simulink model "wave_2"  (Simulink 7.4)
settings: Solver=ode23tb  StartTime=0.0  StopTime=.5  RelTol=1e-3
PreLoadFcn:
  | load gauss_fir;  % pulse shaping coefficients
InitFcn:
  | Ts=1e-4;    % set this to control simulation speed, mainly for wave visualization
  | Line_Length=.05; % in meters
libraries: powerlib x209, simulink x2, dspsrcs4 x1
(part 1 of 2)
settings Model: Creator=Dick  LastModifiedBy=Dick
settings SolverCC: SolverResetMethod=Robust
settings DebuggingCC: SolverPrmCheckMsg=none

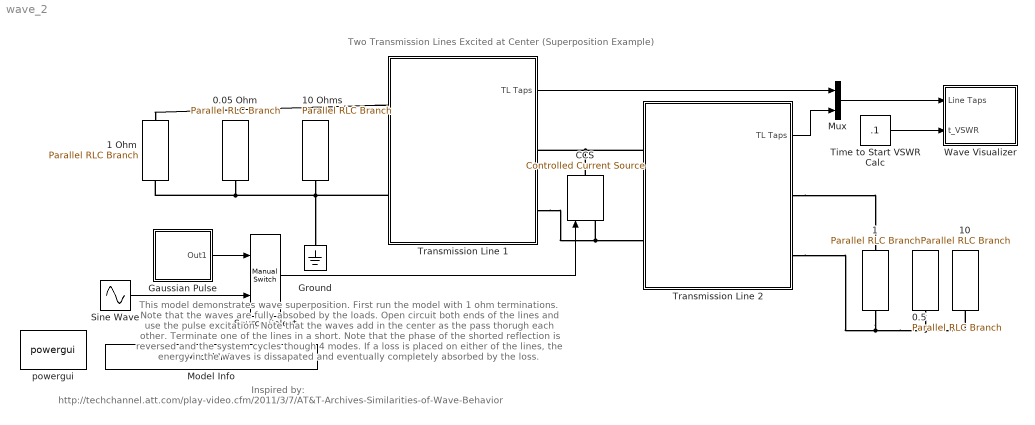
== system wave_2 ==
  note: Two Transmission Lines Excited at Center (Superposition Example)
  note: Inspired by: http://techchannel.att.com/play-video.cfm/2011/3/7/AT&T-Archives-Similarities-of-Wave-Behavior
  note: This model demonstrates wave superposition. First run the model with 1 ohm terminations. Note that the
      | waves are fully absobed by the loads. Open circuit both ends of the lines and use the pulse excitation.
      | Note that the waves add in the center as the pass thorugh each other.
      | Terminate one of the lines in a short. Note that the phase of the shorted reflection
      | is reversed and the system cycles though 4 modes. If a loss is placed on either of the lines,
      | the energy in the waves is dissapated and eventually completely absorbed by the loss.
  0.05 Ohm : powerlib/Elements/Parallel RLC Branch  DialogController=POWERSYS.PowerSysDialog  PhysicalDomain=powersysdomain  SubClassName=unknown  LeftPortType=p1  RightPortType=p1  LConnTagsString=a  RConnTagsString=__new0  BranchType=R  Resistance=.05  Inductance=1e-3  SetiL0=off  InitialCurrent=0  Capacitance=1  Setx0=off  InitialVoltage=0  Measurements=None
  0.5 : powerlib/Elements/Parallel RLC Branch  DialogController=POWERSYS.PowerSysDialog  PhysicalDomain=powersysdomain  SubClassName=unknown  LeftPortType=p1  RightPortType=p1  LConnTagsString=a  RConnTagsString=__new0  BranchType=R  Resistance=.05  Inductance=1e-3  SetiL0=off  InitialCurrent=0  Capacitance=1  Setx0=off  InitialVoltage=0  Measurements=None
  1 : powerlib/Elements/Parallel RLC Branch  DialogController=POWERSYS.PowerSysDialog  PhysicalDomain=powersysdomain  SubClassName=unknown  LeftPortType=p1  RightPortType=p1  LConnTagsString=a  RConnTagsString=__new0  BranchType=R  Resistance=1  Inductance=1e-3  SetiL0=off  InitialCurrent=0  Capacitance=1  Setx0=off  InitialVoltage=0  Measurements=None
  1 Ohm : powerlib/Elements/Parallel RLC Branch  DialogController=POWERSYS.PowerSysDialog  PhysicalDomain=powersysdomain  SubClassName=unknown  LeftPortType=p1  RightPortType=p1  LConnTagsString=a  RConnTagsString=__new0  BranchType=R  Resistance=1  Inductance=1e-3  SetiL0=off  InitialCurrent=0  Capacitance=1  Setx0=off  InitialVoltage=0  Measurements=None
  10 : powerlib/Elements/Parallel RLC Branch  DialogController=POWERSYS.PowerSysDialog  PhysicalDomain=powersysdomain  SubClassName=unknown  LeftPortType=p1  RightPortType=p1  LConnTagsString=a  RConnTagsString=__new0  BranchType=R  Resistance=10  Inductance=1e-3  SetiL0=off  InitialCurrent=0  Capacitance=1  Setx0=off  InitialVoltage=0  Measurements=None
  10 Ohms : powerlib/Elements/Parallel RLC Branch  DialogController=POWERSYS.PowerSysDialog  PhysicalDomain=powersysdomain  SubClassName=unknown  LeftPortType=p1  RightPortType=p1  LConnTagsString=a  RConnTagsString=__new0  BranchType=R  Resistance=10  Inductance=1e-3  SetiL0=off  InitialCurrent=0  Capacitance=1  Setx0=off  InitialVoltage=0  Measurements=None
  CCS : powerlib/Electrical Sources/Controlled Current Source  DialogController=POWERSYS.PowerSysDialog  SystemSampleTime=-1  Initialize=off  Source_Type=DC  Amplitude=0  Phase=0  Frequency=0  Measurements=None
  Gaussian Pulse : Subsystem
  Ground : powerlib/Elements/Ground  DialogController=POWERSYS.PowerSysDialog  PhysicalDomain=powersysdomain  SubClassName=unknown  LeftPortType=p1  RightPortType=p1  LConnTagsString=a
  Model Info : simulink/Model-Wide Utilities/Model Info  SystemSampleTime=-1  InitialBlockCM=None  BlockCM=None  Frame=on  DisplayStringWithTags=Copyright 2012 The MathWorks, Inc.  HorizontalTextAlignment=Center  LeftAlignmentValue=0.5  SourceBlockDiagram=wave_2  TagMaxNumber=20
  Mux : Mux  Inputs=2
  Sine Wave : Sin  Amplitude=1  Bias=0  Frequency=40*2*pi  Phase=0  Samples=10  SampleTime=Ts  Offset=0
  Source Select : simulink/Signal Routing/Manual Switch  SystemSampleTime=-1  sw=0  action=0  varsize=off
  Time to Start VSWR Calc : Constant  Value=.1  OutDataType=fixdt(1, 16)  OutScaling=2^0
  Transmission Line 1 : Subsystem  mask{Zo=1, Vp=1, Len=Line_Length}
      mask prompts: Zo "Zo in ohms"; Vp "Vp in meters/sec"; Len "Line Length in meters"
      mask init:
      | C_1 = ones(1,10)/(Vp*Zo);  % farads/meter
      | L_1 = ones(1,10)*Zo/Vp;    % henrys/meter
      mask CallbackString:
      | % C_1 = ones(1,10)/(Vp*Zo);  % farads/meter
      | % L_1 = ones(1,10)*Zo/Vp;    % henrys/meter
      | |%C_1 = ones(1,10)/(Vp*Zo);  % farads/meter
      | % L_1 = ones(1,10)*Zo/Vp;    % henrys/meter
      | |
      mask Display:
      | disp(['50 Tap Uniform\n Transmission Line \n\n',...
      |        'Zo=',num2str(Zo),' Ohms, \nVp=',num2str(Vp),'m/sec \n',...
      |        'Length=',num2str(Len),' meters'])
  Transmission Line 2 : Subsystem  mask{Zo=1, Vp=1, Len=Line_Length}
      mask prompts: Zo "Zo in ohms"; Vp "Vp in meters/sec"; Len "Line Length in meters"
      mask init:
      | C_1 = ones(1,10)/(Vp*Zo);  % farads/meter
      | L_1 = ones(1,10)*Zo/Vp;    % henrys/meter
      mask CallbackString:
      | % C_1 = ones(1,10)/(Vp*Zo);  % farads/meter
      | % L_1 = ones(1,10)*Zo/Vp;    % henrys/meter
      | |%C_1 = ones(1,10)/(Vp*Zo);  % farads/meter
      | % L_1 = ones(1,10)*Zo/Vp;    % henrys/meter
      | |
      mask Display:
      | disp(['50 Tap Uniform\n Transmission Line \n\n',...
      |        'Zo=',num2str(Zo),' Ohms, \nVp=',num2str(Vp),'m/sec \n',...
      |        'Length=',num2str(Len),' meters'])
  "Wave Visualizer " : Subsystem
  powergui : powerlib/powergui  Priority=1  SystemSampleTime=-1  SimulationMode=Continuous  SampleTime=50e-6  frequency=60  SPID=off  DisableSnubberDevices=off  DisableRonSwitches=off  DisableVfSwitches=off  SwTol=0  Interpol=off  frequencyindice=0  echomessages=off  HookPort=off  DisplayEquations=off  FunctionMessages=off  EnableUseOfTLC=off  x0status=blocks  RestoreLinks=warning  Frange=[0:2:500]  Ylog=off  Xlog=on  ShowGrid=off  save=off  variable=ZData  ZoomFFT=on  StartTime=0.0  cycles=1  DisplayStyle=1  fundamental=60  FreqAxis=off  MaxFrequency=1000  frequencyindicesteady=1  RmsSteady=1  display=off  Ts=0  methode=off
  wires:
  Sine Wave/1 -> Source Select/2
  Gaussian Pulse/1(Out1) -> Source Select/1
  Mux/1 -> "Wave Visualizer "/1(Line Taps)
  Transmission Line 1/1(TL Taps) -> Mux/1
  Transmission Line 2/1(TL Taps) -> Mux/2
  Time to Start VSWR Calc/1 -> "Wave Visualizer "/2(t_VSWR)
  Source Select/1 -> CCS/1
  connections:
  Transmission Line 1/LConn2 -- 0.05 Ohm/RConn1 -- 1 Ohm/RConn1 -- 10 Ohms/RConn1 -- Ground/LConn1
  Transmission Line 2/RConn2 -- 10/RConn1 -- 0.5/RConn1 -- 1/RConn1
  Transmission Line 2/LConn1 -- Transmission Line 1/RConn1 -- CCS/RConn1
  Transmission Line 1/RConn2 -- Transmission Line 2/LConn2 -- CCS/LConn1
  Transmission Line 1/LConn1 -- 1 Ohm/LConn1
  Transmission Line 2/RConn1 -- 1/LConn1

== system wave_2/Gaussian Pulse ==
  Discrete  Impulse : dspsrcs4/Discrete  Impulse  Delay=0  SampleTime=Ts  FrameSample=1  dataType=double  isSigned=on  wordLen=16  udDataType=sfix(16)  fracBitsMode=Best precision  numFracBits=15
  Discrete FIR Filter : DiscreteFir  NumCoeffs=h_gauss
  Out1 : Outport
  wires:
  Discrete  Impulse/1 -> Discrete FIR Filter/1
  Discrete FIR Filter/1 -> Out1/1

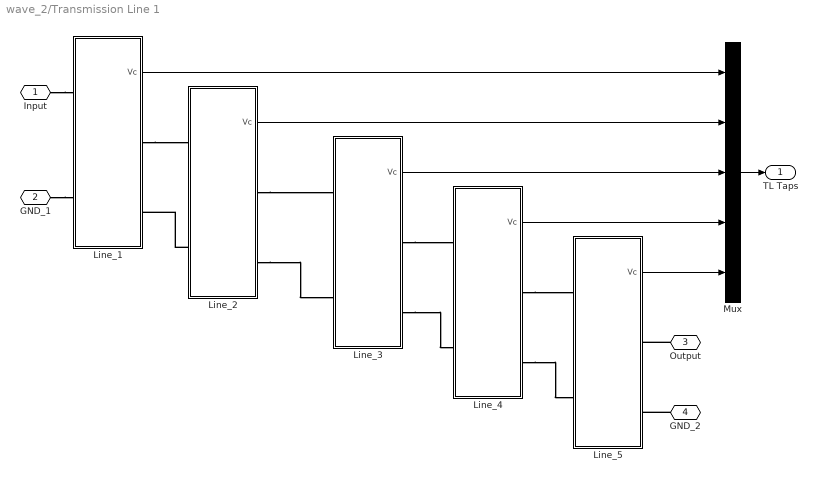
== system wave_2/Transmission Line 1 ==
  Line_1 : Subsystem  mask{R=zeros(1,10), L=L_1, C=C_1, Len=Len/5}
      mask prompts: R "Rvector(1:10) ohms/meter"; L "Lvector(1:10) henrys/meter"; C "Cvector(1:10) farards/meter"; Len "Length in m"
      mask Display: disp('TRL Section')
  Line_2 : Subsystem  mask{R=zeros(1,10), L=L_1, C=C_1, Len=Len/5}
      mask prompts: R "Rvector(1:10) ohms/meter"; L "Lvector(1:10) henrys/meter"; C "Cvector(1:10) farards/meter"; Len "Length in m"
      mask Display: disp('TRL Section')
  Line_3 : Subsystem  mask{R=zeros(1,10), L=L_1, C=C_1, Len=Len/5}
      mask prompts: R "Rvector(1:10) ohms/meter"; L "Lvector(1:10) henrys/meter"; C "Cvector(1:10) farards/meter"; Len "Length in m"
      mask Display: disp('TRL Section')
  Line_4 : Subsystem  mask{R=zeros(1,10), L=L_1, C=C_1, Len=Len/5}
      mask prompts: R "Rvector(1:10) ohms/meter"; L "Lvector(1:10) henrys/meter"; C "Cvector(1:10) farards/meter"; Len "Length in m"
      mask Display: disp('TRL Section')
  Line_5 : Subsystem  mask{R=zeros(1,10), L=L_1, C=C_1, Len=Len/5}
      mask prompts: R "Rvector(1:10) ohms/meter"; L "Lvector(1:10) henrys/meter"; C "Cvector(1:10) farards/meter"; Len "Length in m"
      mask Display: disp('TRL Section')
  Mux : Mux  Inputs=5
  Input : PMIOPort  Port=1  Side=Left
  GND_1 : PMIOPort  Port=2  Side=Left
  Output : PMIOPort  Port=3  Side=Right
  GND_2 : PMIOPort  Port=4  Side=Right
  TL Taps : Outport
  wires:
  Line_1/1(Vc) -> Mux/1
  Line_2/1(Vc) -> Mux/2
  Line_5/1(Vc) -> Mux/5
  Line_3/1(Vc) -> Mux/3
  Line_4/1(Vc) -> Mux/4
  Mux/1 -> TL Taps/1
  connections:
  Line_1/RConn1 -- Line_2/LConn1
  Line_2/LConn2 -- Line_1/RConn2
  Line_2/RConn1 -- Line_3/LConn1
  Line_2/RConn2 -- Line_3/LConn2
  Line_3/RConn1 -- Line_4/LConn1
  Line_3/RConn2 -- Line_4/LConn2
  Line_4/RConn1 -- Line_5/LConn1
  Line_4/RConn2 -- Line_5/LConn2
  Input/RConn1 -- Line_1/LConn1
  GND_1/RConn1 -- Line_1/LConn2
  Output/RConn1 -- Line_5/RConn1
  GND_2/RConn1 -- Line_5/RConn2

== system wave_2/Transmission Line 2 ==
  Line_1 : Subsystem  mask{R=zeros(1,10), L=L_1, C=C_1, Len=Len/5}
      mask prompts: R "Rvector(1:10) ohms/meter"; L "Lvector(1:10) henrys/meter"; C "Cvector(1:10) farards/meter"; Len "Length in m"
      mask Display: disp('TRL Section')
  Line_2 : Subsystem  mask{R=zeros(1,10), L=L_1, C=C_1, Len=Len/5}
      mask prompts: R "Rvector(1:10) ohms/meter"; L "Lvector(1:10) henrys/meter"; C "Cvector(1:10) farards/meter"; Len "Length in m"
      mask Display: disp('TRL Section')
  Line_3 : Subsystem  mask{R=zeros(1,10), L=L_1, C=C_1, Len=Len/5}
      mask prompts: R "Rvector(1:10) ohms/meter"; L "Lvector(1:10) henrys/meter"; C "Cvector(1:10) farards/meter"; Len "Length in m"
      mask Display: disp('TRL Section')
  Line_4 : Subsystem  mask{R=zeros(1,10), L=L_1, C=C_1, Len=Len/5}
      mask prompts: R "Rvector(1:10) ohms/meter"; L "Lvector(1:10) henrys/meter"; C "Cvector(1:10) farards/meter"; Len "Length in m"
      mask Display: disp('TRL Section')
  Line_5 : Subsystem  mask{R=zeros(1,10), L=L_1, C=C_1, Len=Len/5}
      mask prompts: R "Rvector(1:10) ohms/meter"; L "Lvector(1:10) henrys/meter"; C "Cvector(1:10) farards/meter"; Len "Length in m"
      mask Display: disp('TRL Section')
  Mux : Mux  Inputs=5
  Input : PMIOPort  Port=1  Side=Left
  GND_1 : PMIOPort  Port=2  Side=Left
  Output : PMIOPort  Port=3  Side=Right
  GND_2 : PMIOPort  Port=4  Side=Right
  TL Taps : Outport
  wires:
  Mux/1 -> TL Taps/1
  Line_4/1(Vc) -> Mux/4
  Line_3/1(Vc) -> Mux/3
  Line_5/1(Vc) -> Mux/5
  Line_2/1(Vc) -> Mux/2
  Line_1/1(Vc) -> Mux/1
  connections:
  GND_2/RConn1 -- Line_5/RConn2
  Output/RConn1 -- Line_5/RConn1
  GND_1/RConn1 -- Line_1/LConn2
  Input/RConn1 -- Line_1/LConn1
  Line_4/RConn2 -- Line_5/LConn2
  Line_4/RConn1 -- Line_5/LConn1
  Line_3/RConn2 -- Line_4/LConn2
  Line_3/RConn1 -- Line_4/LConn1
  Line_2/RConn2 -- Line_3/LConn2
  Line_2/RConn1 -- Line_3/LConn1
  Line_2/LConn2 -- Line_1/RConn2
  Line_1/RConn1 -- Line_2/LConn1

== system wave_2/Wave Visualizer  ==
  note: The VSWR calculaltion uses the maximum and minimum values of the PEAK of the wave over the simulation run.
      | Therefore, the transmision line system needs to have achieved steady state conditions before the calculation is started.
      | This time will vary with line configurations as well as source and load terminations. Ther VSWR is measured on Line 1.
      | Obviously the sine source must be used.
  Line Taps : Inport
  t_VSWR : Inport  Port=2
  Clock : Clock
  Constant3 : Constant  Value=Line_Length  OutDataType=fixdt(1, 16)  OutScaling=2^0  SampleTime=Ts
  Line  Section Tap  Voltage : Stateflow chart
  Zero-Order Hold : ZeroOrderHold  SampleTime=Ts
  Zero-Order Hold1 : ZeroOrderHold  SampleTime=Ts
  wires:
  Zero-Order Hold/1 -> Line  Section Tap  Voltage/1(y)
  Constant3/1 -> Line  Section Tap  Voltage/3(Line_Length)
  Clock/1 -> Zero-Order Hold1/1
  Zero-Order Hold1/1 -> Line  Section Tap  Voltage/2(t)
  Line Taps/1 -> Zero-Order Hold/1
  t_VSWR/1 -> Line  Section Tap  Voltage/4(t_VSWR)

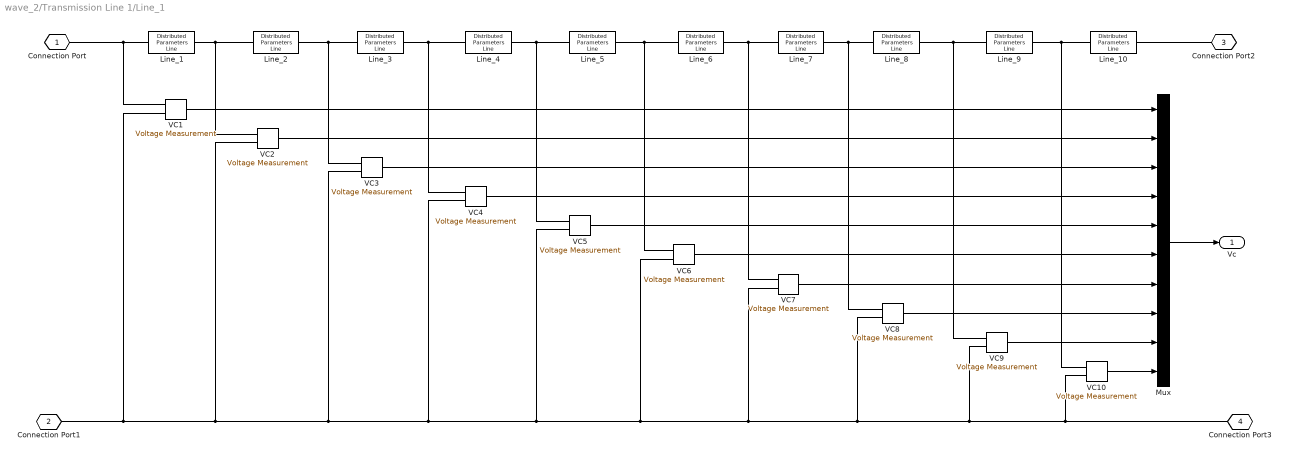
== system wave_2/Transmission Line 1/Line_1 ==
  Line_1 : powerlib/Elements/Distributed Parameters Line  DialogController=POWERSYS.PowerSysDialog  SystemSampleTime=-1  Phases=1  Frequency=60  Resistance=R(1)*1000  Inductance=L(1)*1000  Capacitance=C(1)*1000  Length=Len/(10*1000); % 10 sections in this subsystem  x1=[0 0;0.0002 0;0.0004 0;0.0006 0;0.0008 0;0.001 0]  x2=[0 0;0.0002 0;0.0004 0;0.0006 0;0.0008 0;0.001 0]  x3=[0 0;0.0002 0;0.0004 0;0.0006 0;0.0008 0;0.001 0]  x4=[0 0;0.0002 0;0.0004 0;0.0006 0;0.0008 0;0.001 0]  x5=0.001  Measurements=None
  Line_10 : powerlib/Elements/Distributed Parameters Line  DialogController=POWERSYS.PowerSysDialog  SystemSampleTime=-1  Phases=1  Frequency=60  Resistance=R(10)*1000  Inductance=L(10)*1000  Capacitance=C(10)*1000  Length=Len/(10*1000); % 10 sections in this subsystem  x1=[0 0;0.0002 0;0.0004 0;0.0006 0;0.0008 0;0.001 0]  x2=[0 0;0.0002 0;0.0004 0;0.0006 0;0.0008 0;0.001 0]  x3=[0 0;0.0002 0;0.0004 0;0.0006 0;0.0008 0;0.001 0]  x4=[0 0;0.0002 0;0.0004 0;0.0006 0;0.0008 0;0.001 0]  x5=0.001  Measurements=None
  Line_2 : powerlib/Elements/Distributed Parameters Line  DialogController=POWERSYS.PowerSysDialog  SystemSampleTime=-1  Phases=1  Frequency=60  Resistance=R(2)*1000  Inductance=L(2)*1000  Capacitance=C(2)*1000  Length=Len/(10*1000); % 10 sections in this subsystem  x1=[0 0;0.0002 0;0.0004 0;0.0006 0;0.0008 0;0.001 0]  x2=[0 0;0.0002 0;0.0004 0;0.0006 0;0.0008 0;0.001 0]  x3=[0 0;0.0002 0;0.0004 0;0.0006 0;0.0008 0;0.001 0]  x4=[0 0;0.0002 0;0.0004 0;0.0006 0;0.0008 0;0.001 0]  x5=0.001  Measurements=None
  Line_3 : powerlib/Elements/Distributed Parameters Line  DialogController=POWERSYS.PowerSysDialog  SystemSampleTime=-1  Phases=1  Frequency=60  Resistance=R(3)*1000  Inductance=L(3)*1000  Capacitance=C(3)*1000  Length=Len/(10*1000); % 10 sections in this subsystem  x1=[0 0;0.0002 0;0.0004 0;0.0006 0;0.0008 0;0.001 0]  x2=[0 0;0.0002 0;0.0004 0;0.0006 0;0.0008 0;0.001 0]  x3=[0 0;0.0002 0;0.0004 0;0.0006 0;0.0008 0;0.001 0]  x4=[0 0;0.0002 0;0.0004 0;0.0006 0;0.0008 0;0.001 0]  x5=0.001  Measurements=None
  Line_4 : powerlib/Elements/Distributed Parameters Line  DialogController=POWERSYS.PowerSysDialog  SystemSampleTime=-1  Phases=1  Frequency=60  Resistance=R(4)*1000  Inductance=L(4)*1000  Capacitance=C(4)*1000  Length=Len/(10*1000); % 10 sections in this subsystem  x1=[0 0;0.0002 0;0.0004 0;0.0006 0;0.0008 0;0.001 0]  x2=[0 0;0.0002 0;0.0004 0;0.0006 0;0.0008 0;0.001 0]  x3=[0 0;0.0002 0;0.0004 0;0.0006 0;0.0008 0;0.001 0]  x4=[0 0;0.0002 0;0.0004 0;0.0006 0;0.0008 0;0.001 0]  x5=0.001  Measurements=None
  Line_5 : powerlib/Elements/Distributed Parameters Line  DialogController=POWERSYS.PowerSysDialog  SystemSampleTime=-1  Phases=1  Frequency=60  Resistance=R(5)*1000  Inductance=L(5)*1000  Capacitance=C(5)*1000  Length=Len/(10*1000); % 10 sections in this subsystem  x1=[0 0;0.0002 0;0.0004 0;0.0006 0;0.0008 0;0.001 0]  x2=[0 0;0.0002 0;0.0004 0;0.0006 0;0.0008 0;0.001 0]  x3=[0 0;0.0002 0;0.0004 0;0.0006 0;0.0008 0;0.001 0]  x4=[0 0;0.0002 0;0.0004 0;0.0006 0;0.0008 0;0.001 0]  x5=0.001  Measurements=None
  Line_6 : powerlib/Elements/Distributed Parameters Line  DialogController=POWERSYS.PowerSysDialog  SystemSampleTime=-1  Phases=1  Frequency=60  Resistance=R(6)*1000  Inductance=L(6)*1000  Capacitance=C(6)*1000  Length=Len/(10*1000); % 10 sections in this subsystem  x1=[0 0;0.0002 0;0.0004 0;0.0006 0;0.0008 0;0.001 0]  x2=[0 0;0.0002 0;0.0004 0;0.0006 0;0.0008 0;0.001 0]  x3=[0 0;0.0002 0;0.0004 0;0.0006 0;0.0008 0;0.001 0]  x4=[0 0;0.0002 0;0.0004 0;0.0006 0;0.0008 0;0.001 0]  x5=0.001  Measurements=None
  Line_7 : powerlib/Elements/Distributed Parameters Line  DialogController=POWERSYS.PowerSysDialog  SystemSampleTime=-1  Phases=1  Frequency=60  Resistance=R(7)*1000  Inductance=L(7)*1000  Capacitance=C(7)*1000  Length=Len/(10*1000); % 10 sections in this subsystem  x1=[0 0;0.0002 0;0.0004 0;0.0006 0;0.0008 0;0.001 0]  x2=[0 0;0.0002 0;0.0004 0;0.0006 0;0.0008 0;0.001 0]  x3=[0 0;0.0002 0;0.0004 0;0.0006 0;0.0008 0;0.001 0]  x4=[0 0;0.0002 0;0.0004 0;0.0006 0;0.0008 0;0.001 0]  x5=0.001  Measurements=None
  Line_8 : powerlib/Elements/Distributed Parameters Line  DialogController=POWERSYS.PowerSysDialog  SystemSampleTime=-1  Phases=1  Frequency=60  Resistance=R(8)*1000  Inductance=L(8)*1000  Capacitance=C(8)*1000  Length=Len/(10*1000); % 10 sections in this subsystem  x1=[0 0;0.0002 0;0.0004 0;0.0006 0;0.0008 0;0.001 0]  x2=[0 0;0.0002 0;0.0004 0;0.0006 0;0.0008 0;0.001 0]  x3=[0 0;0.0002 0;0.0004 0;0.0006 0;0.0008 0;0.001 0]  x4=[0 0;0.0002 0;0.0004 0;0.0006 0;0.0008 0;0.001 0]  x5=0.001  Measurements=None
  Line_9 : powerlib/Elements/Distributed Parameters Line  DialogController=POWERSYS.PowerSysDialog  SystemSampleTime=-1  Phases=1  Frequency=60  Resistance=R(9)*1000  Inductance=L(9)*1000  Capacitance=C(9)*1000  Length=Len/(10*1000); % 10 sections in this subsystem  x1=[0 0;0.0002 0;0.0004 0;0.0006 0;0.0008 0;0.001 0]  x2=[0 0;0.0002 0;0.0004 0;0.0006 0;0.0008 0;0.001 0]  x3=[0 0;0.0002 0;0.0004 0;0.0006 0;0.0008 0;0.001 0]  x4=[0 0;0.0002 0;0.0004 0;0.0006 0;0.0008 0;0.001 0]  x5=0.001  Measurements=None
  Mux : Mux  Inputs=10
  VC{1..10} (10 alike) : powerlib/Measurements/Voltage Measurement  DialogController=POWERSYS.PowerSysDialog  SystemSampleTime=-1  PhasorSimulation=off  OutputType=Complex  PSBequivalent=0
  Connection Port : PMIOPort  Tag=PMCPort  Port=1  Side=Left
  Connection Port1 : PMIOPort  Tag=PMCPort  Port=2  Side=Left
  Connection Port2 : PMIOPort  Tag=PMCPort  Port=3  Side=Right
  Connection Port3 : PMIOPort  Tag=PMCPort  Port=4  Side=Right
  Vc : Outport  OutDataType=fixdt(1, 16)  OutScaling=2^0
  wires:
  VC1/1 -> Mux/1
  VC10/1 -> Mux/10
  VC9/1 -> Mux/9
  VC8/1 -> Mux/8
  VC7/1 -> Mux/7
  VC6/1 -> Mux/6
  VC5/1 -> Mux/5
  VC4/1 -> Mux/4
  VC3/1 -> Mux/3
  VC2/1 -> Mux/2
  Mux/1 -> Vc/1
  connections:
  Connection Port1/RConn1 -- Connection Port3/RConn1 -- VC10/LConn2 -- VC9/LConn2 -- VC8/LConn2 -- VC7/LConn2 -- VC6/LConn2 -- VC5/LConn2 -- VC4/LConn2 -- VC3/LConn2 -- VC2/LConn2 -- VC1/LConn2
  Line_10/RConn1 -- Connection Port2/RConn1
  Connection Port/RConn1 -- Line_1/LConn1 -- VC1/LConn1
  Line_1/RConn1 -- Line_2/LConn1 -- VC2/LConn1
  Line_2/RConn1 -- Line_3/LConn1 -- VC3/LConn1
  Line_3/RConn1 -- Line_4/LConn1 -- VC4/LConn1
  Line_4/RConn1 -- Line_5/LConn1 -- VC5/LConn1
  Line_5/RConn1 -- Line_6/LConn1 -- VC6/LConn1
  Line_6/RConn1 -- Line_7/LConn1 -- VC7/LConn1
  Line_7/RConn1 -- Line_8/LConn1 -- VC8/LConn1
  Line_8/RConn1 -- Line_9/LConn1 -- VC9/LConn1
  Line_9/RConn1 -- Line_10/LConn1 -- VC10/LConn1

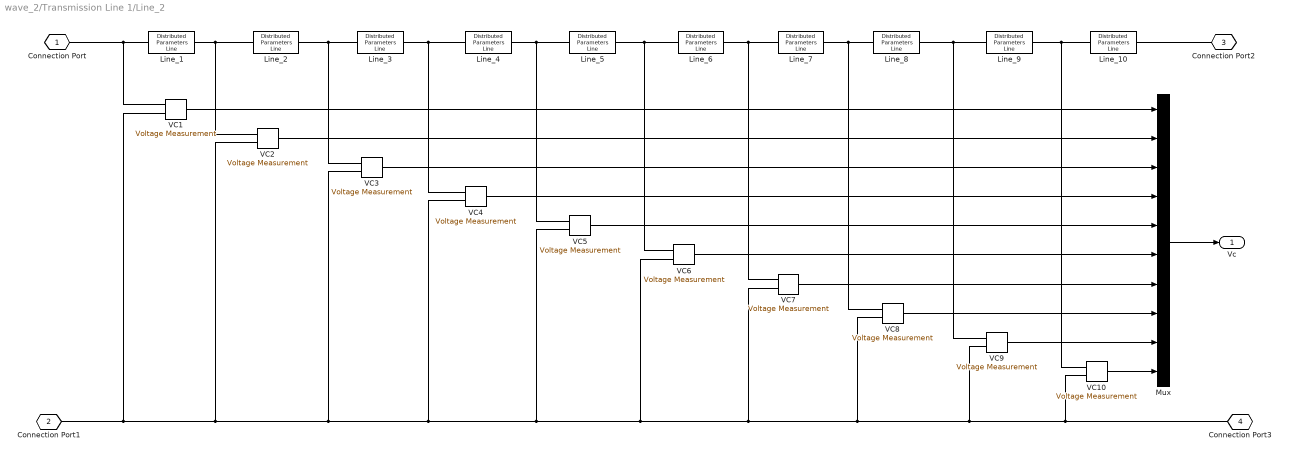
== system wave_2/Transmission Line 1/Line_2 ==
  Line_1 : powerlib/Elements/Distributed Parameters Line  DialogController=POWERSYS.PowerSysDialog  SystemSampleTime=-1  Phases=1  Frequency=60  Resistance=R(1)*1000  Inductance=L(1)*1000  Capacitance=C(1)*1000  Length=Len/(10*1000); % 10 sections in this subsystem  x1=[0 0;0.0002 0;0.0004 0;0.0006 0;0.0008 0;0.001 0]  x2=[0 0;0.0002 0;0.0004 0;0.0006 0;0.0008 0;0.001 0]  x3=[0 0;0.0002 0;0.0004 0;0.0006 0;0.0008 0;0.001 0]  x4=[0 0;0.0002 0;0.0004 0;0.0006 0;0.0008 0;0.001 0]  x5=0.001  Measurements=None
  Line_10 : powerlib/Elements/Distributed Parameters Line  DialogController=POWERSYS.PowerSysDialog  SystemSampleTime=-1  Phases=1  Frequency=60  Resistance=R(10)*1000  Inductance=L(10)*1000  Capacitance=C(10)*1000  Length=Len/(10*1000); % 10 sections in this subsystem  x1=[0 0;0.0002 0;0.0004 0;0.0006 0;0.0008 0;0.001 0]  x2=[0 0;0.0002 0;0.0004 0;0.0006 0;0.0008 0;0.001 0]  x3=[0 0;0.0002 0;0.0004 0;0.0006 0;0.0008 0;0.001 0]  x4=[0 0;0.0002 0;0.0004 0;0.0006 0;0.0008 0;0.001 0]  x5=0.001  Measurements=None
  Line_2 : powerlib/Elements/Distributed Parameters Line  DialogController=POWERSYS.PowerSysDialog  SystemSampleTime=-1  Phases=1  Frequency=60  Resistance=R(2)*1000  Inductance=L(2)*1000  Capacitance=C(2)*1000  Length=Len/(10*1000); % 10 sections in this subsystem  x1=[0 0;0.0002 0;0.0004 0;0.0006 0;0.0008 0;0.001 0]  x2=[0 0;0.0002 0;0.0004 0;0.0006 0;0.0008 0;0.001 0]  x3=[0 0;0.0002 0;0.0004 0;0.0006 0;0.0008 0;0.001 0]  x4=[0 0;0.0002 0;0.0004 0;0.0006 0;0.0008 0;0.001 0]  x5=0.001  Measurements=None
  Line_3 : powerlib/Elements/Distributed Parameters Line  DialogController=POWERSYS.PowerSysDialog  SystemSampleTime=-1  Phases=1  Frequency=60  Resistance=R(3)*1000  Inductance=L(3)*1000  Capacitance=C(3)*1000  Length=Len/(10*1000); % 10 sections in this subsystem  x1=[0 0;0.0002 0;0.0004 0;0.0006 0;0.0008 0;0.001 0]  x2=[0 0;0.0002 0;0.0004 0;0.0006 0;0.0008 0;0.001 0]  x3=[0 0;0.0002 0;0.0004 0;0.0006 0;0.0008 0;0.001 0]  x4=[0 0;0.0002 0;0.0004 0;0.0006 0;0.0008 0;0.001 0]  x5=0.001  Measurements=None
  Line_4 : powerlib/Elements/Distributed Parameters Line  DialogController=POWERSYS.PowerSysDialog  SystemSampleTime=-1  Phases=1  Frequency=60  Resistance=R(4)*1000  Inductance=L(4)*1000  Capacitance=C(4)*1000  Length=Len/(10*1000); % 10 sections in this subsystem  x1=[0 0;0.0002 0;0.0004 0;0.0006 0;0.0008 0;0.001 0]  x2=[0 0;0.0002 0;0.0004 0;0.0006 0;0.0008 0;0.001 0]  x3=[0 0;0.0002 0;0.0004 0;0.0006 0;0.0008 0;0.001 0]  x4=[0 0;0.0002 0;0.0004 0;0.0006 0;0.0008 0;0.001 0]  x5=0.001  Measurements=None
  Line_5 : powerlib/Elements/Distributed Parameters Line  DialogController=POWERSYS.PowerSysDialog  SystemSampleTime=-1  Phases=1  Frequency=60  Resistance=R(5)*1000  Inductance=L(5)*1000  Capacitance=C(5)*1000  Length=Len/(10*1000); % 10 sections in this subsystem  x1=[0 0;0.0002 0;0.0004 0;0.0006 0;0.0008 0;0.001 0]  x2=[0 0;0.0002 0;0.0004 0;0.0006 0;0.0008 0;0.001 0]  x3=[0 0;0.0002 0;0.0004 0;0.0006 0;0.0008 0;0.001 0]  x4=[0 0;0.0002 0;0.0004 0;0.0006 0;0.0008 0;0.001 0]  x5=0.001  Measurements=None
  Line_6 : powerlib/Elements/Distributed Parameters Line  DialogController=POWERSYS.PowerSysDialog  SystemSampleTime=-1  Phases=1  Frequency=60  Resistance=R(6)*1000  Inductance=L(6)*1000  Capacitance=C(6)*1000  Length=Len/(10*1000); % 10 sections in this subsystem  x1=[0 0;0.0002 0;0.0004 0;0.0006 0;0.0008 0;0.001 0]  x2=[0 0;0.0002 0;0.0004 0;0.0006 0;0.0008 0;0.001 0]  x3=[0 0;0.0002 0;0.0004 0;0.0006 0;0.0008 0;0.001 0]  x4=[0 0;0.0002 0;0.0004 0;0.0006 0;0.0008 0;0.001 0]  x5=0.001  Measurements=None
  Line_7 : powerlib/Elements/Distributed Parameters Line  DialogController=POWERSYS.PowerSysDialog  SystemSampleTime=-1  Phases=1  Frequency=60  Resistance=R(7)*1000  Inductance=L(7)*1000  Capacitance=C(7)*1000  Length=Len/(10*1000); % 10 sections in this subsystem  x1=[0 0;0.0002 0;0.0004 0;0.0006 0;0.0008 0;0.001 0]  x2=[0 0;0.0002 0;0.0004 0;0.0006 0;0.0008 0;0.001 0]  x3=[0 0;0.0002 0;0.0004 0;0.0006 0;0.0008 0;0.001 0]  x4=[0 0;0.0002 0;0.0004 0;0.0006 0;0.0008 0;0.001 0]  x5=0.001  Measurements=None
  Line_8 : powerlib/Elements/Distributed Parameters Line  DialogController=POWERSYS.PowerSysDialog  SystemSampleTime=-1  Phases=1  Frequency=60  Resistance=R(8)*1000  Inductance=L(8)*1000  Capacitance=C(8)*1000  Length=Len/(10*1000); % 10 sections in this subsystem  x1=[0 0;0.0002 0;0.0004 0;0.0006 0;0.0008 0;0.001 0]  x2=[0 0;0.0002 0;0.0004 0;0.0006 0;0.0008 0;0.001 0]  x3=[0 0;0.0002 0;0.0004 0;0.0006 0;0.0008 0;0.001 0]  x4=[0 0;0.0002 0;0.0004 0;0.0006 0;0.0008 0;0.001 0]  x5=0.001  Measurements=None
  Line_9 : powerlib/Elements/Distributed Parameters Line  DialogController=POWERSYS.PowerSysDialog  SystemSampleTime=-1  Phases=1  Frequency=60  Resistance=R(9)*1000  Inductance=L(9)*1000  Capacitance=C(9)*1000  Length=Len/(10*1000); % 10 sections in this subsystem  x1=[0 0;0.0002 0;0.0004 0;0.0006 0;0.0008 0;0.001 0]  x2=[0 0;0.0002 0;0.0004 0;0.0006 0;0.0008 0;0.001 0]  x3=[0 0;0.0002 0;0.0004 0;0.0006 0;0.0008 0;0.001 0]  x4=[0 0;0.0002 0;0.0004 0;0.0006 0;0.0008 0;0.001 0]  x5=0.001  Measurements=None
  Mux : Mux  Inputs=10
  VC{1..10} (10 alike) : powerlib/Measurements/Voltage Measurement  DialogController=POWERSYS.PowerSysDialog  SystemSampleTime=-1  PhasorSimulation=off  OutputType=Complex  PSBequivalent=0
  Connection Port : PMIOPort  Tag=PMCPort  Port=1  Side=Left
  Connection Port1 : PMIOPort  Tag=PMCPort  Port=2  Side=Left
  Connection Port2 : PMIOPort  Tag=PMCPort  Port=3  Side=Right
  Connection Port3 : PMIOPort  Tag=PMCPort  Port=4  Side=Right
  Vc : Outport  OutDataType=fixdt(1, 16)  OutScaling=2^0
  wires:
  Mux/1 -> Vc/1
  VC2/1 -> Mux/2
  VC3/1 -> Mux/3
  VC4/1 -> Mux/4
  VC5/1 -> Mux/5
  VC6/1 -> Mux/6
  VC7/1 -> Mux/7
  VC8/1 -> Mux/8
  VC9/1 -> Mux/9
  VC10/1 -> Mux/10
  VC1/1 -> Mux/1
  connections:
  VC10/LConn1 -- Line_10/LConn1 -- Line_9/RConn1
  VC9/LConn1 -- Line_9/LConn1 -- Line_8/RConn1
  VC8/LConn1 -- Line_8/LConn1 -- Line_7/RConn1
  VC7/LConn1 -- Line_7/LConn1 -- Line_6/RConn1
  VC6/LConn1 -- Line_6/LConn1 -- Line_5/RConn1
  VC5/LConn1 -- Line_5/LConn1 -- Line_4/RConn1
  VC4/LConn1 -- Line_4/LConn1 -- Line_3/RConn1
  VC3/LConn1 -- Line_3/LConn1 -- Line_2/RConn1
  VC2/LConn1 -- Line_2/LConn1 -- Line_1/RConn1
  VC1/LConn1 -- Line_1/LConn1 -- Connection Port/RConn1
  Line_10/RConn1 -- Connection Port2/RConn1
  VC1/LConn2 -- VC2/LConn2 -- VC3/LConn2 -- VC4/LConn2 -- VC5/LConn2 -- VC6/LConn2 -- VC7/LConn2 -- VC8/LConn2 -- VC9/LConn2 -- VC10/LConn2 -- Connection Port3/RConn1 -- Connection Port1/RConn1

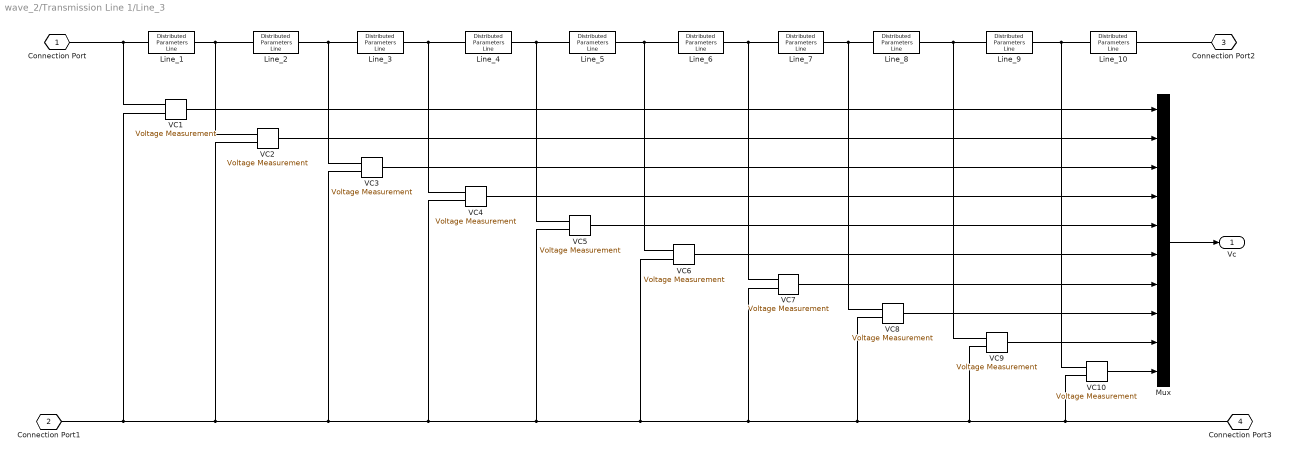
== system wave_2/Transmission Line 1/Line_3 ==
  Line_1 : powerlib/Elements/Distributed Parameters Line  DialogController=POWERSYS.PowerSysDialog  SystemSampleTime=-1  Phases=1  Frequency=60  Resistance=R(1)*1000  Inductance=L(1)*1000  Capacitance=C(1)*1000  Length=Len/(10*1000); % 10 sections in this subsystem  x1=[0 0;0.0002 0;0.0004 0;0.0006 0;0.0008 0;0.001 0]  x2=[0 0;0.0002 0;0.0004 0;0.0006 0;0.0008 0;0.001 0]  x3=[0 0;0.0002 0;0.0004 0;0.0006 0;0.0008 0;0.001 0]  x4=[0 0;0.0002 0;0.0004 0;0.0006 0;0.0008 0;0.001 0]  x5=0.001  Measurements=None
  Line_10 : powerlib/Elements/Distributed Parameters Line  DialogController=POWERSYS.PowerSysDialog  SystemSampleTime=-1  Phases=1  Frequency=60  Resistance=R(10)*1000  Inductance=L(10)*1000  Capacitance=C(10)*1000  Length=Len/(10*1000); % 10 sections in this subsystem  x1=[0 0;0.0002 0;0.0004 0;0.0006 0;0.0008 0;0.001 0]  x2=[0 0;0.0002 0;0.0004 0;0.0006 0;0.0008 0;0.001 0]  x3=[0 0;0.0002 0;0.0004 0;0.0006 0;0.0008 0;0.001 0]  x4=[0 0;0.0002 0;0.0004 0;0.0006 0;0.0008 0;0.001 0]  x5=0.001  Measurements=None
  Line_2 : powerlib/Elements/Distributed Parameters Line  DialogController=POWERSYS.PowerSysDialog  SystemSampleTime=-1  Phases=1  Frequency=60  Resistance=R(2)*1000  Inductance=L(2)*1000  Capacitance=C(2)*1000  Length=Len/(10*1000); % 10 sections in this subsystem  x1=[0 0;0.0002 0;0.0004 0;0.0006 0;0.0008 0;0.001 0]  x2=[0 0;0.0002 0;0.0004 0;0.0006 0;0.0008 0;0.001 0]  x3=[0 0;0.0002 0;0.0004 0;0.0006 0;0.0008 0;0.001 0]  x4=[0 0;0.0002 0;0.0004 0;0.0006 0;0.0008 0;0.001 0]  x5=0.001  Measurements=None
  Line_3 : powerlib/Elements/Distributed Parameters Line  DialogController=POWERSYS.PowerSysDialog  SystemSampleTime=-1  Phases=1  Frequency=60  Resistance=R(3)*1000  Inductance=L(3)*1000  Capacitance=C(3)*1000  Length=Len/(10*1000); % 10 sections in this subsystem  x1=[0 0;0.0002 0;0.0004 0;0.0006 0;0.0008 0;0.001 0]  x2=[0 0;0.0002 0;0.0004 0;0.0006 0;0.0008 0;0.001 0]  x3=[0 0;0.0002 0;0.0004 0;0.0006 0;0.0008 0;0.001 0]  x4=[0 0;0.0002 0;0.0004 0;0.0006 0;0.0008 0;0.001 0]  x5=0.001  Measurements=None
  Line_4 : powerlib/Elements/Distributed Parameters Line  DialogController=POWERSYS.PowerSysDialog  SystemSampleTime=-1  Phases=1  Frequency=60  Resistance=R(4)*1000  Inductance=L(4)*1000  Capacitance=C(4)*1000  Length=Len/(10*1000); % 10 sections in this subsystem  x1=[0 0;0.0002 0;0.0004 0;0.0006 0;0.0008 0;0.001 0]  x2=[0 0;0.0002 0;0.0004 0;0.0006 0;0.0008 0;0.001 0]  x3=[0 0;0.0002 0;0.0004 0;0.0006 0;0.0008 0;0.001 0]  x4=[0 0;0.0002 0;0.0004 0;0.0006 0;0.0008 0;0.001 0]  x5=0.001  Measurements=None
  Line_5 : powerlib/Elements/Distributed Parameters Line  DialogController=POWERSYS.PowerSysDialog  SystemSampleTime=-1  Phases=1  Frequency=60  Resistance=R(5)*1000  Inductance=L(5)*1000  Capacitance=C(5)*1000  Length=Len/(10*1000); % 10 sections in this subsystem  x1=[0 0;0.0002 0;0.0004 0;0.0006 0;0.0008 0;0.001 0]  x2=[0 0;0.0002 0;0.0004 0;0.0006 0;0.0008 0;0.001 0]  x3=[0 0;0.0002 0;0.0004 0;0.0006 0;0.0008 0;0.001 0]  x4=[0 0;0.0002 0;0.0004 0;0.0006 0;0.0008 0;0.001 0]  x5=0.001  Measurements=None
  Line_6 : powerlib/Elements/Distributed Parameters Line  DialogController=POWERSYS.PowerSysDialog  SystemSampleTime=-1  Phases=1  Frequency=60  Resistance=R(6)*1000  Inductance=L(6)*1000  Capacitance=C(6)*1000  Length=Len/(10*1000); % 10 sections in this subsystem  x1=[0 0;0.0002 0;0.0004 0;0.0006 0;0.0008 0;0.001 0]  x2=[0 0;0.0002 0;0.0004 0;0.0006 0;0.0008 0;0.001 0]  x3=[0 0;0.0002 0;0.0004 0;0.0006 0;0.0008 0;0.001 0]  x4=[0 0;0.0002 0;0.0004 0;0.0006 0;0.0008 0;0.001 0]  x5=0.001  Measurements=None
  Line_7 : powerlib/Elements/Distributed Parameters Line  DialogController=POWERSYS.PowerSysDialog  SystemSampleTime=-1  Phases=1  Frequency=60  Resistance=R(7)*1000  Inductance=L(7)*1000  Capacitance=C(7)*1000  Length=Len/(10*1000); % 10 sections in this subsystem  x1=[0 0;0.0002 0;0.0004 0;0.0006 0;0.0008 0;0.001 0]  x2=[0 0;0.0002 0;0.0004 0;0.0006 0;0.0008 0;0.001 0]  x3=[0 0;0.0002 0;0.0004 0;0.0006 0;0.0008 0;0.001 0]  x4=[0 0;0.0002 0;0.0004 0;0.0006 0;0.0008 0;0.001 0]  x5=0.001  Measurements=None
  Line_8 : powerlib/Elements/Distributed Parameters Line  DialogController=POWERSYS.PowerSysDialog  SystemSampleTime=-1  Phases=1  Frequency=60  Resistance=R(8)*1000  Inductance=L(8)*1000  Capacitance=C(8)*1000  Length=Len/(10*1000); % 10 sections in this subsystem  x1=[0 0;0.0002 0;0.0004 0;0.0006 0;0.0008 0;0.001 0]  x2=[0 0;0.0002 0;0.0004 0;0.0006 0;0.0008 0;0.001 0]  x3=[0 0;0.0002 0;0.0004 0;0.0006 0;0.0008 0;0.001 0]  x4=[0 0;0.0002 0;0.0004 0;0.0006 0;0.0008 0;0.001 0]  x5=0.001  Measurements=None
  Line_9 : powerlib/Elements/Distributed Parameters Line  DialogController=POWERSYS.PowerSysDialog  SystemSampleTime=-1  Phases=1  Frequency=60  Resistance=R(9)*1000  Inductance=L(9)*1000  Capacitance=C(9)*1000  Length=Len/(10*1000); % 10 sections in this subsystem  x1=[0 0;0.0002 0;0.0004 0;0.0006 0;0.0008 0;0.001 0]  x2=[0 0;0.0002 0;0.0004 0;0.0006 0;0.0008 0;0.001 0]  x3=[0 0;0.0002 0;0.0004 0;0.0006 0;0.0008 0;0.001 0]  x4=[0 0;0.0002 0;0.0004 0;0.0006 0;0.0008 0;0.001 0]  x5=0.001  Measurements=None
  Mux : Mux  Inputs=10
  VC{1..10} (10 alike) : powerlib/Measurements/Voltage Measurement  DialogController=POWERSYS.PowerSysDialog  SystemSampleTime=-1  PhasorSimulation=off  OutputType=Complex  PSBequivalent=0
  Connection Port : PMIOPort  Tag=PMCPort  Port=1  Side=Left
  Connection Port1 : PMIOPort  Tag=PMCPort  Port=2  Side=Left
  Connection Port2 : PMIOPort  Tag=PMCPort  Port=3  Side=Right
  Connection Port3 : PMIOPort  Tag=PMCPort  Port=4  Side=Right
  Vc : Outport  OutDataType=fixdt(1, 16)  OutScaling=2^0
  wires:
  VC1/1 -> Mux/1
  VC10/1 -> Mux/10
  VC9/1 -> Mux/9
  VC8/1 -> Mux/8
  VC7/1 -> Mux/7
  VC6/1 -> Mux/6
  VC5/1 -> Mux/5
  VC4/1 -> Mux/4
  VC3/1 -> Mux/3
  VC2/1 -> Mux/2
  Mux/1 -> Vc/1
  connections:
  Connection Port1/RConn1 -- Connection Port3/RConn1 -- VC10/LConn2 -- VC9/LConn2 -- VC8/LConn2 -- VC7/LConn2 -- VC6/LConn2 -- VC5/LConn2 -- VC4/LConn2 -- VC3/LConn2 -- VC2/LConn2 -- VC1/LConn2
  Line_10/RConn1 -- Connection Port2/RConn1
  Connection Port/RConn1 -- Line_1/LConn1 -- VC1/LConn1
  Line_1/RConn1 -- Line_2/LConn1 -- VC2/LConn1
  Line_2/RConn1 -- Line_3/LConn1 -- VC3/LConn1
  Line_3/RConn1 -- Line_4/LConn1 -- VC4/LConn1
  Line_4/RConn1 -- Line_5/LConn1 -- VC5/LConn1
  Line_5/RConn1 -- Line_6/LConn1 -- VC6/LConn1
  Line_6/RConn1 -- Line_7/LConn1 -- VC7/LConn1
  Line_7/RConn1 -- Line_8/LConn1 -- VC8/LConn1
  Line_8/RConn1 -- Line_9/LConn1 -- VC9/LConn1
  Line_9/RConn1 -- Line_10/LConn1 -- VC10/LConn1

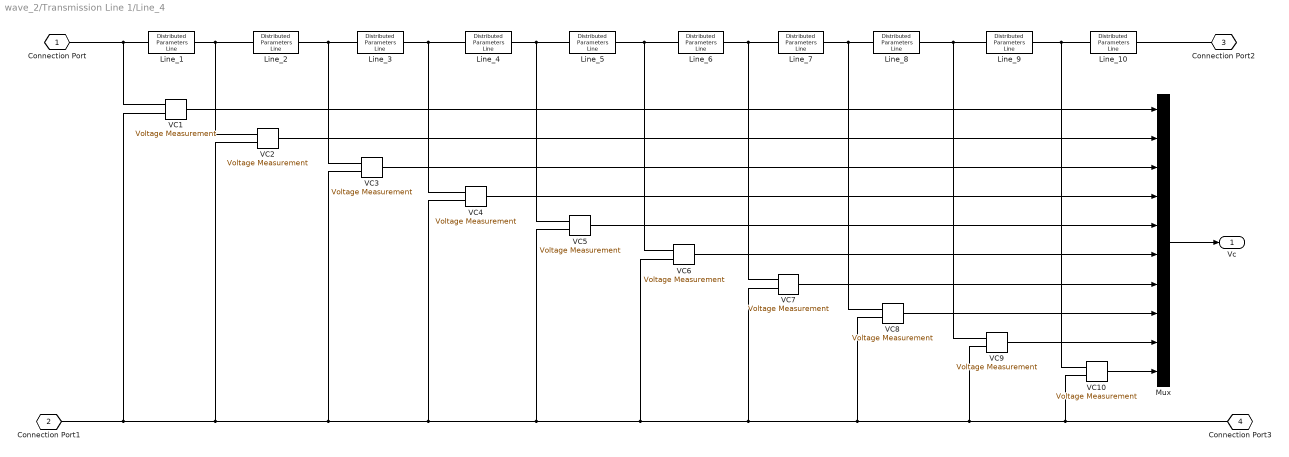
== system wave_2/Transmission Line 1/Line_4 ==
  Line_1 : powerlib/Elements/Distributed Parameters Line  DialogController=POWERSYS.PowerSysDialog  SystemSampleTime=-1  Phases=1  Frequency=60  Resistance=R(1)*1000  Inductance=L(1)*1000  Capacitance=C(1)*1000  Length=Len/(10*1000); % 10 sections in this subsystem  x1=[0 0;0.0002 0;0.0004 0;0.0006 0;0.0008 0;0.001 0]  x2=[0 0;0.0002 0;0.0004 0;0.0006 0;0.0008 0;0.001 0]  x3=[0 0;0.0002 0;0.0004 0;0.0006 0;0.0008 0;0.001 0]  x4=[0 0;0.0002 0;0.0004 0;0.0006 0;0.0008 0;0.001 0]  x5=0.001  Measurements=None
  Line_10 : powerlib/Elements/Distributed Parameters Line  DialogController=POWERSYS.PowerSysDialog  SystemSampleTime=-1  Phases=1  Frequency=60  Resistance=R(10)*1000  Inductance=L(10)*1000  Capacitance=C(10)*1000  Length=Len/(10*1000); % 10 sections in this subsystem  x1=[0 0;0.0002 0;0.0004 0;0.0006 0;0.0008 0;0.001 0]  x2=[0 0;0.0002 0;0.0004 0;0.0006 0;0.0008 0;0.001 0]  x3=[0 0;0.0002 0;0.0004 0;0.0006 0;0.0008 0;0.001 0]  x4=[0 0;0.0002 0;0.0004 0;0.0006 0;0.0008 0;0.001 0]  x5=0.001  Measurements=None
  Line_2 : powerlib/Elements/Distributed Parameters Line  DialogController=POWERSYS.PowerSysDialog  SystemSampleTime=-1  Phases=1  Frequency=60  Resistance=R(2)*1000  Inductance=L(2)*1000  Capacitance=C(2)*1000  Length=Len/(10*1000); % 10 sections in this subsystem  x1=[0 0;0.0002 0;0.0004 0;0.0006 0;0.0008 0;0.001 0]  x2=[0 0;0.0002 0;0.0004 0;0.0006 0;0.0008 0;0.001 0]  x3=[0 0;0.0002 0;0.0004 0;0.0006 0;0.0008 0;0.001 0]  x4=[0 0;0.0002 0;0.0004 0;0.0006 0;0.0008 0;0.001 0]  x5=0.001  Measurements=None
  Line_3 : powerlib/Elements/Distributed Parameters Line  DialogController=POWERSYS.PowerSysDialog  SystemSampleTime=-1  Phases=1  Frequency=60  Resistance=R(3)*1000  Inductance=L(3)*1000  Capacitance=C(3)*1000  Length=Len/(10*1000); % 10 sections in this subsystem  x1=[0 0;0.0002 0;0.0004 0;0.0006 0;0.0008 0;0.001 0]  x2=[0 0;0.0002 0;0.0004 0;0.0006 0;0.0008 0;0.001 0]  x3=[0 0;0.0002 0;0.0004 0;0.0006 0;0.0008 0;0.001 0]  x4=[0 0;0.0002 0;0.0004 0;0.0006 0;0.0008 0;0.001 0]  x5=0.001  Measurements=None
  Line_4 : powerlib/Elements/Distributed Parameters Line  DialogController=POWERSYS.PowerSysDialog  SystemSampleTime=-1  Phases=1  Frequency=60  Resistance=R(4)*1000  Inductance=L(4)*1000  Capacitance=C(4)*1000  Length=Len/(10*1000); % 10 sections in this subsystem  x1=[0 0;0.0002 0;0.0004 0;0.0006 0;0.0008 0;0.001 0]  x2=[0 0;0.0002 0;0.0004 0;0.0006 0;0.0008 0;0.001 0]  x3=[0 0;0.0002 0;0.0004 0;0.0006 0;0.0008 0;0.001 0]  x4=[0 0;0.0002 0;0.0004 0;0.0006 0;0.0008 0;0.001 0]  x5=0.001  Measurements=None
  Line_5 : powerlib/Elements/Distributed Parameters Line  DialogController=POWERSYS.PowerSysDialog  SystemSampleTime=-1  Phases=1  Frequency=60  Resistance=R(5)*1000  Inductance=L(5)*1000  Capacitance=C(5)*1000  Length=Len/(10*1000); % 10 sections in this subsystem  x1=[0 0;0.0002 0;0.0004 0;0.0006 0;0.0008 0;0.001 0]  x2=[0 0;0.0002 0;0.0004 0;0.0006 0;0.0008 0;0.001 0]  x3=[0 0;0.0002 0;0.0004 0;0.0006 0;0.0008 0;0.001 0]  x4=[0 0;0.0002 0;0.0004 0;0.0006 0;0.0008 0;0.001 0]  x5=0.001  Measurements=None
  Line_6 : powerlib/Elements/Distributed Parameters Line  DialogController=POWERSYS.PowerSysDialog  SystemSampleTime=-1  Phases=1  Frequency=60  Resistance=R(6)*1000  Inductance=L(6)*1000  Capacitance=C(6)*1000  Length=Len/(10*1000); % 10 sections in this subsystem  x1=[0 0;0.0002 0;0.0004 0;0.0006 0;0.0008 0;0.001 0]  x2=[0 0;0.0002 0;0.0004 0;0.0006 0;0.0008 0;0.001 0]  x3=[0 0;0.0002 0;0.0004 0;0.0006 0;0.0008 0;0.001 0]  x4=[0 0;0.0002 0;0.0004 0;0.0006 0;0.0008 0;0.001 0]  x5=0.001  Measurements=None
  Line_7 : powerlib/Elements/Distributed Parameters Line  DialogController=POWERSYS.PowerSysDialog  SystemSampleTime=-1  Phases=1  Frequency=60  Resistance=R(7)*1000  Inductance=L(7)*1000  Capacitance=C(7)*1000  Length=Len/(10*1000); % 10 sections in this subsystem  x1=[0 0;0.0002 0;0.0004 0;0.0006 0;0.0008 0;0.001 0]  x2=[0 0;0.0002 0;0.0004 0;0.0006 0;0.0008 0;0.001 0]  x3=[0 0;0.0002 0;0.0004 0;0.0006 0;0.0008 0;0.001 0]  x4=[0 0;0.0002 0;0.0004 0;0.0006 0;0.0008 0;0.001 0]  x5=0.001  Measurements=None
  Line_8 : powerlib/Elements/Distributed Parameters Line  DialogController=POWERSYS.PowerSysDialog  SystemSampleTime=-1  Phases=1  Frequency=60  Resistance=R(8)*1000  Inductance=L(8)*1000  Capacitance=C(8)*1000  Length=Len/(10*1000); % 10 sections in this subsystem  x1=[0 0;0.0002 0;0.0004 0;0.0006 0;0.0008 0;0.001 0]  x2=[0 0;0.0002 0;0.0004 0;0.0006 0;0.0008 0;0.001 0]  x3=[0 0;0.0002 0;0.0004 0;0.0006 0;0.0008 0;0.001 0]  x4=[0 0;0.0002 0;0.0004 0;0.0006 0;0.0008 0;0.001 0]  x5=0.001  Measurements=None
  Line_9 : powerlib/Elements/Distributed Parameters Line  DialogController=POWERSYS.PowerSysDialog  SystemSampleTime=-1  Phases=1  Frequency=60  Resistance=R(9)*1000  Inductance=L(9)*1000  Capacitance=C(9)*1000  Length=Len/(10*1000); % 10 sections in this subsystem  x1=[0 0;0.0002 0;0.0004 0;0.0006 0;0.0008 0;0.001 0]  x2=[0 0;0.0002 0;0.0004 0;0.0006 0;0.0008 0;0.001 0]  x3=[0 0;0.0002 0;0.0004 0;0.0006 0;0.0008 0;0.001 0]  x4=[0 0;0.0002 0;0.0004 0;0.0006 0;0.0008 0;0.001 0]  x5=0.001  Measurements=None
  Mux : Mux  Inputs=10
  VC{1..10} (10 alike) : powerlib/Measurements/Voltage Measurement  DialogController=POWERSYS.PowerSysDialog  SystemSampleTime=-1  PhasorSimulation=off  OutputType=Complex  PSBequivalent=0
  Connection Port : PMIOPort  Tag=PMCPort  Port=1  Side=Left
  Connection Port1 : PMIOPort  Tag=PMCPort  Port=2  Side=Left
  Connection Port2 : PMIOPort  Tag=PMCPort  Port=3  Side=Right
  Connection Port3 : PMIOPort  Tag=PMCPort  Port=4  Side=Right
  Vc : Outport  OutDataType=fixdt(1, 16)  OutScaling=2^0
  wires:
  Mux/1 -> Vc/1
  VC2/1 -> Mux/2
  VC3/1 -> Mux/3
  VC4/1 -> Mux/4
  VC5/1 -> Mux/5
  VC6/1 -> Mux/6
  VC7/1 -> Mux/7
  VC8/1 -> Mux/8
  VC9/1 -> Mux/9
  VC10/1 -> Mux/10
  VC1/1 -> Mux/1
  connections:
  VC10/LConn1 -- Line_10/LConn1 -- Line_9/RConn1
  VC9/LConn1 -- Line_9/LConn1 -- Line_8/RConn1
  VC8/LConn1 -- Line_8/LConn1 -- Line_7/RConn1
  VC7/LConn1 -- Line_7/LConn1 -- Line_6/RConn1
  VC6/LConn1 -- Line_6/LConn1 -- Line_5/RConn1
  VC5/LConn1 -- Line_5/LConn1 -- Line_4/RConn1
  VC4/LConn1 -- Line_4/LConn1 -- Line_3/RConn1
  VC3/LConn1 -- Line_3/LConn1 -- Line_2/RConn1
  VC2/LConn1 -- Line_2/LConn1 -- Line_1/RConn1
  VC1/LConn1 -- Line_1/LConn1 -- Connection Port/RConn1
  Line_10/RConn1 -- Connection Port2/RConn1
  VC1/LConn2 -- VC2/LConn2 -- VC3/LConn2 -- VC4/LConn2 -- VC5/LConn2 -- VC6/LConn2 -- VC7/LConn2 -- VC8/LConn2 -- VC9/LConn2 -- VC10/LConn2 -- Connection Port3/RConn1 -- Connection Port1/RConn1

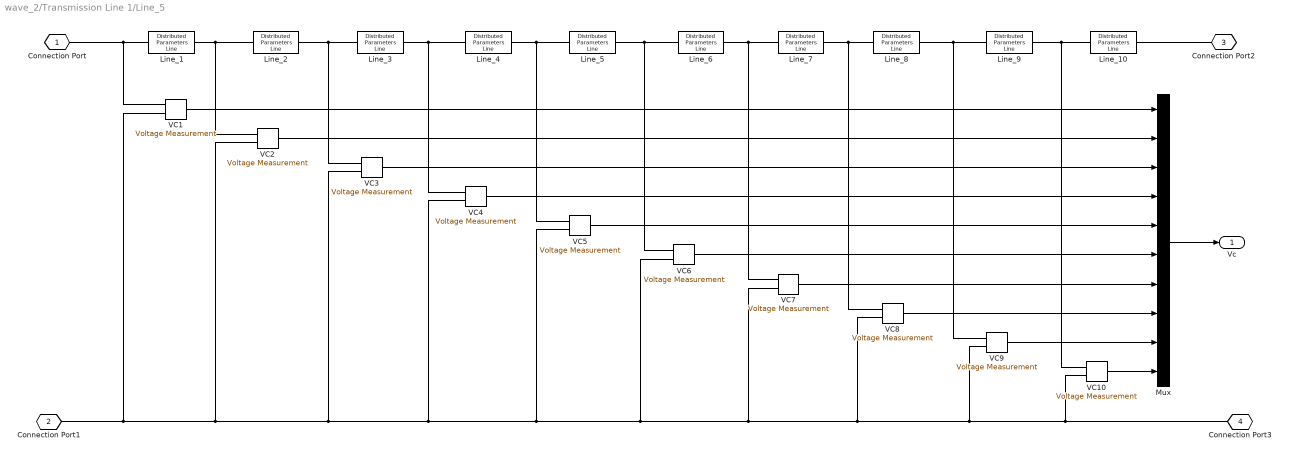
== system wave_2/Transmission Line 1/Line_5 ==
  Line_1 : powerlib/Elements/Distributed Parameters Line  DialogController=POWERSYS.PowerSysDialog  SystemSampleTime=-1  Phases=1  Frequency=60  Resistance=R(1)*1000  Inductance=L(1)*1000  Capacitance=C(1)*1000  Length=Len/(10*1000); % 10 sections in this subsystem  x1=[0 0;0.0002 0;0.0004 0;0.0006 0;0.0008 0;0.001 0]  x2=[0 0;0.0002 0;0.0004 0;0.0006 0;0.0008 0;0.001 0]  x3=[0 0;0.0002 0;0.0004 0;0.0006 0;0.0008 0;0.001 0]  x4=[0 0;0.0002 0;0.0004 0;0.0006 0;0.0008 0;0.001 0]  x5=0.001  Measurements=None
  Line_10 : powerlib/Elements/Distributed Parameters Line  DialogController=POWERSYS.PowerSysDialog  SystemSampleTime=-1  Phases=1  Frequency=60  Resistance=R(10)*1000  Inductance=L(10)*1000  Capacitance=C(10)*1000  Length=Len/(10*1000); % 10 sections in this subsystem  x1=[0 0;0.0002 0;0.0004 0;0.0006 0;0.0008 0;0.001 0]  x2=[0 0;0.0002 0;0.0004 0;0.0006 0;0.0008 0;0.001 0]  x3=[0 0;0.0002 0;0.0004 0;0.0006 0;0.0008 0;0.001 0]  x4=[0 0;0.0002 0;0.0004 0;0.0006 0;0.0008 0;0.001 0]  x5=0.001  Measurements=None
  Line_2 : powerlib/Elements/Distributed Parameters Line  DialogController=POWERSYS.PowerSysDialog  SystemSampleTime=-1  Phases=1  Frequency=60  Resistance=R(2)*1000  Inductance=L(2)*1000  Capacitance=C(2)*1000  Length=Len/(10*1000); % 10 sections in this subsystem  x1=[0 0;0.0002 0;0.0004 0;0.0006 0;0.0008 0;0.001 0]  x2=[0 0;0.0002 0;0.0004 0;0.0006 0;0.0008 0;0.001 0]  x3=[0 0;0.0002 0;0.0004 0;0.0006 0;0.0008 0;0.001 0]  x4=[0 0;0.0002 0;0.0004 0;0.0006 0;0.0008 0;0.001 0]  x5=0.001  Measurements=None
  Line_3 : powerlib/Elements/Distributed Parameters Line  DialogController=POWERSYS.PowerSysDialog  SystemSampleTime=-1  Phases=1  Frequency=60  Resistance=R(3)*1000  Inductance=L(3)*1000  Capacitance=C(3)*1000  Length=Len/(10*1000); % 10 sections in this subsystem  x1=[0 0;0.0002 0;0.0004 0;0.0006 0;0.0008 0;0.001 0]  x2=[0 0;0.0002 0;0.0004 0;0.0006 0;0.0008 0;0.001 0]  x3=[0 0;0.0002 0;0.0004 0;0.0006 0;0.0008 0;0.001 0]  x4=[0 0;0.0002 0;0.0004 0;0.0006 0;0.0008 0;0.001 0]  x5=0.001  Measurements=None
  Line_4 : powerlib/Elements/Distributed Parameters Line  DialogController=POWERSYS.PowerSysDialog  SystemSampleTime=-1  Phases=1  Frequency=60  Resistance=R(4)*1000  Inductance=L(4)*1000  Capacitance=C(4)*1000  Length=Len/(10*1000); % 10 sections in this subsystem  x1=[0 0;0.0002 0;0.0004 0;0.0006 0;0.0008 0;0.001 0]  x2=[0 0;0.0002 0;0.0004 0;0.0006 0;0.0008 0;0.001 0]  x3=[0 0;0.0002 0;0.0004 0;0.0006 0;0.0008 0;0.001 0]  x4=[0 0;0.0002 0;0.0004 0;0.0006 0;0.0008 0;0.001 0]  x5=0.001  Measurements=None
  Line_5 : powerlib/Elements/Distributed Parameters Line  DialogController=POWERSYS.PowerSysDialog  SystemSampleTime=-1  Phases=1  Frequency=60  Resistance=R(5)*1000  Inductance=L(5)*1000  Capacitance=C(5)*1000  Length=Len/(10*1000); % 10 sections in this subsystem  x1=[0 0;0.0002 0;0.0004 0;0.0006 0;0.0008 0;0.001 0]  x2=[0 0;0.0002 0;0.0004 0;0.0006 0;0.0008 0;0.001 0]  x3=[0 0;0.0002 0;0.0004 0;0.0006 0;0.0008 0;0.001 0]  x4=[0 0;0.0002 0;0.0004 0;0.0006 0;0.0008 0;0.001 0]  x5=0.001  Measurements=None
  Line_6 : powerlib/Elements/Distributed Parameters Line  DialogController=POWERSYS.PowerSysDialog  SystemSampleTime=-1  Phases=1  Frequency=60  Resistance=R(6)*1000  Inductance=L(6)*1000  Capacitance=C(6)*1000  Length=Len/(10*1000); % 10 sections in this subsystem  x1=[0 0;0.0002 0;0.0004 0;0.0006 0;0.0008 0;0.001 0]  x2=[0 0;0.0002 0;0.0004 0;0.0006 0;0.0008 0;0.001 0]  x3=[0 0;0.0002 0;0.0004 0;0.0006 0;0.0008 0;0.001 0]  x4=[0 0;0.0002 0;0.0004 0;0.0006 0;0.0008 0;0.001 0]  x5=0.001  Measurements=None
  Line_7 : powerlib/Elements/Distributed Parameters Line  DialogController=POWERSYS.PowerSysDialog  SystemSampleTime=-1  Phases=1  Frequency=60  Resistance=R(7)*1000  Inductance=L(7)*1000  Capacitance=C(7)*1000  Length=Len/(10*1000); % 10 sections in this subsystem  x1=[0 0;0.0002 0;0.0004 0;0.0006 0;0.0008 0;0.001 0]  x2=[0 0;0.0002 0;0.0004 0;0.0006 0;0.0008 0;0.001 0]  x3=[0 0;0.0002 0;0.0004 0;0.0006 0;0.0008 0;0.001 0]  x4=[0 0;0.0002 0;0.0004 0;0.0006 0;0.0008 0;0.001 0]  x5=0.001  Measurements=None
  Line_8 : powerlib/Elements/Distributed Parameters Line  DialogController=POWERSYS.PowerSysDialog  SystemSampleTime=-1  Phases=1  Frequency=60  Resistance=R(8)*1000  Inductance=L(8)*1000  Capacitance=C(8)*1000  Length=Len/(10*1000); % 10 sections in this subsystem  x1=[0 0;0.0002 0;0.0004 0;0.0006 0;0.0008 0;0.001 0]  x2=[0 0;0.0002 0;0.0004 0;0.0006 0;0.0008 0;0.001 0]  x3=[0 0;0.0002 0;0.0004 0;0.0006 0;0.0008 0;0.001 0]  x4=[0 0;0.0002 0;0.0004 0;0.0006 0;0.0008 0;0.001 0]  x5=0.001  Measurements=None
  Line_9 : powerlib/Elements/Distributed Parameters Line  DialogController=POWERSYS.PowerSysDialog  SystemSampleTime=-1  Phases=1  Frequency=60  Resistance=R(9)*1000  Inductance=L(9)*1000  Capacitance=C(9)*1000  Length=Len/(10*1000); % 10 sections in this subsystem  x1=[0 0;0.0002 0;0.0004 0;0.0006 0;0.0008 0;0.001 0]  x2=[0 0;0.0002 0;0.0004 0;0.0006 0;0.0008 0;0.001 0]  x3=[0 0;0.0002 0;0.0004 0;0.0006 0;0.0008 0;0.001 0]  x4=[0 0;0.0002 0;0.0004 0;0.0006 0;0.0008 0;0.001 0]  x5=0.001  Measurements=None
  Mux : Mux  Inputs=10
  VC{1..10} (10 alike) : powerlib/Measurements/Voltage Measurement  DialogController=POWERSYS.PowerSysDialog  SystemSampleTime=-1  PhasorSimulation=off  OutputType=Complex  PSBequivalent=0
  Connection Port : PMIOPort  Tag=PMCPort  Port=1  Side=Left
  Connection Port1 : PMIOPort  Tag=PMCPort  Port=2  Side=Left
  Connection Port2 : PMIOPort  Tag=PMCPort  Port=3  Side=Right
  Connection Port3 : PMIOPort  Tag=PMCPort  Port=4  Side=Right
  Vc : Outport  OutDataType=fixdt(1, 16)  OutScaling=2^0
  wires:
  VC1/1 -> Mux/1
  VC10/1 -> Mux/10
  VC9/1 -> Mux/9
  VC8/1 -> Mux/8
  VC7/1 -> Mux/7
  VC6/1 -> Mux/6
  VC5/1 -> Mux/5
  VC4/1 -> Mux/4
  VC3/1 -> Mux/3
  VC2/1 -> Mux/2
  Mux/1 -> Vc/1
  connections:
  Connection Port1/RConn1 -- Connection Port3/RConn1 -- VC10/LConn2 -- VC9/LConn2 -- VC8/LConn2 -- VC7/LConn2 -- VC6/LConn2 -- VC5/LConn2 -- VC4/LConn2 -- VC3/LConn2 -- VC2/LConn2 -- VC1/LConn2
  Line_10/RConn1 -- Connection Port2/RConn1
  Connection Port/RConn1 -- Line_1/LConn1 -- VC1/LConn1
  Line_1/RConn1 -- Line_2/LConn1 -- VC2/LConn1
  Line_2/RConn1 -- Line_3/LConn1 -- VC3/LConn1
  Line_3/RConn1 -- Line_4/LConn1 -- VC4/LConn1
  Line_4/RConn1 -- Line_5/LConn1 -- VC5/LConn1
  Line_5/RConn1 -- Line_6/LConn1 -- VC6/LConn1
  Line_6/RConn1 -- Line_7/LConn1 -- VC7/LConn1
  Line_7/RConn1 -- Line_8/LConn1 -- VC8/LConn1
  Line_8/RConn1 -- Line_9/LConn1 -- VC9/LConn1
  Line_9/RConn1 -- Line_10/LConn1 -- VC10/LConn1
